simulink model "suspension_simul"  (R2020a)
settings: Solver=VariableStepAuto  StartTime=0.0  StopTime=50  RelTol=1e-3
values from neighbouring files (symbols this model uses):
  b1 = 350    [suspension.m]
  b2 = 15020    [suspension.m]
  k1 = 80000    [suspension.m]
  k2 = 500000    [suspension.m]
  m1 = 2500    [suspension.m]
  m2 = 320    [suspension.m]
settings Model: Creator=root  LastModifiedBy=root

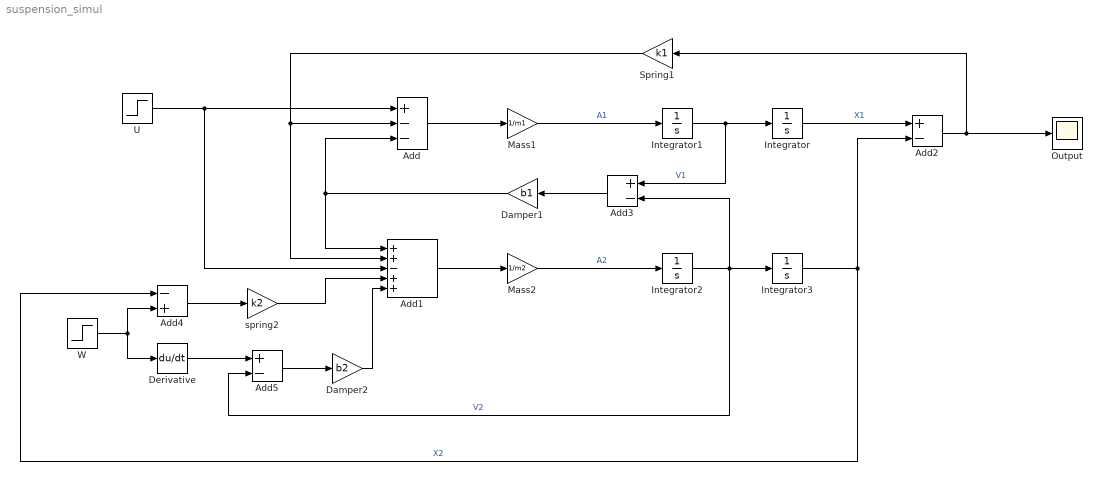
== system suspension_simul ==
  Add : Sum  Inputs=+--
  Add1 : Sum  Inputs=++-++
  Add2 : Sum  Inputs=+-
  Add3 : Sum  Inputs=+-
  Add4 : Sum  Inputs=-+
  Add5 : Sum  Inputs=+-
  Damper1 : Gain  Gain=b1
  Damper2 : Gain  Gain=b2
  Derivative : Derivative
  Integrator{,1..3} (4 alike) : Integrator
  Mass1 : Gain  Gain=1/m1
  Mass2 : Gain  Gain=1/m2
  Output : Scope
  Spring1 : Gain  Gain=k1
  U : Step  Time=0  SampleTime=0
  W : Step  Time=0  After=0  SampleTime=0
  spring2 : Gain  Gain=k2
  wires:
  Integrator1/1 -> Add3/1, Integrator/1  "V1"
  Integrator2/1 -> Add5/2, Integrator3/1, Add3/2  "V2"
  Integrator/1 -> Add2/1  "X1"
  Integrator3/1 -> Add2/2, Add4/1  "X2"
  Mass1/1 -> Integrator1/1  "A1"
  Mass2/1 -> Integrator2/1  "A2"
  Add2/1 -> Output/1, Spring1/1
  Spring1/1 -> Add/2, Add1/2
  Add/1 -> Mass1/1
  Add1/1 -> Mass2/1
  Add3/1 -> Damper1/1
  Damper1/1 -> Add1/1, Add/3
  spring2/1 -> Add1/4
  Add4/1 -> spring2/1
  W/1 -> Add4/2, Derivative/1
  Derivative/1 -> Add5/1
  Add5/1 -> Damper2/1
  Damper2/1 -> Add1/5
  U/1 -> Add/1, Add1/3
